simulink model "PROVA_EGO_ACC_V5"  (R2021b)
settings: Solver=ode4  StartTime=0.0  StopTime=T  FixedStep=Tc  RelTol=1e-3
values from neighbouring files (symbols this model uses):
  acc_C4 = acc_C4_all(i)    [TEST_AUTOMATICO_V1.m]
  acc_C5 = acc_C5_all(i)    [TEST_AUTOMATICO_V1.m]
  init_sim = [X0 (V0_ego_init/3.6) Angles0]'    [TEST_AUTOMATICO_V1.m]
  init_sim_C4 = [X0_C4 (V0_C4_init/3.6) Angles0_C4]'    [TEST_AUTOMATICO_V1.m]
  init_sim_C5 = [X0_C5 (V0_C5_init/3.6) Angles0_C5]'    [TEST_AUTOMATICO_V1.m]
  init_sim_C7 = [X0_C7 (V0_C7_init/3.6) Angles0_C7]'    [TEST_AUTOMATICO_V1.m]
  T = 40    [TEST_AUTOMATICO_V1.m]
  Tc = 0.1    [TEST_AUTOMATICO_V1.m]
  V0_C4_init = V0_C4(i)    [TEST_AUTOMATICO_V1.m]
  V0_C5_init = V0_C5(i)    [TEST_AUTOMATICO_V1.m]
  V0_C7_init = V0_C7(i)    [TEST_AUTOMATICO_V1.m]
  V0_ego_init = V0_ego(i)    [TEST_AUTOMATICO_V1.m]
  xx_rif = 0:Tc:x_tr(end)    [TEST_AUTOMATICO_V1.m]
  xx_rif_C4 = 0:Tc:(x_tr_C4(end))    [TEST_AUTOMATICO_V1.m]
  xx_rif_C5 = 0:Tc:(x_tr_C5(end))    [TEST_AUTOMATICO_V1.m]
  xx_rif_C7 = 0:Tc:(x_tr_C7(end))    [TEST_AUTOMATICO_V1.m]
undefined symbols (not defined in the file or in its folder): yy_rif, yy_rif_C4, yy_rif_C5, yy_rif_C7
libraries: simulink x3, mpcadaslib x2
settings Model: Creator=The MathWorks, Inc.  LastModifiedBy=NICO
settings SolverCC: AlgebraicLoopSolver=TrustRegion
settings DataIOCC: ReturnWorkspaceOutputs=off
settings DebuggingCC: SFMachineParentedDataDiag=warning  ArithmeticOperatorsInVariantConditions=warning
settings SFSimCC: SimUseLocalCustomCode=off  CustomCodeUndefinedFunction=UseInterfaceOnly
settings RTWCC: RTWUseLocalCustomCode=off
settings CodeAppCC: StateflowObjectComments=on

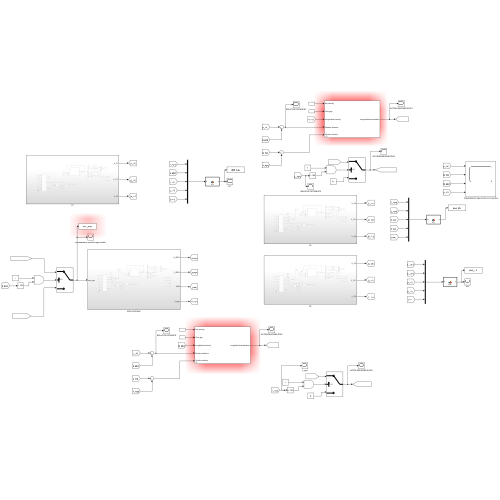
[thumbnail: Simulink's stored preview of the top-level diagram]
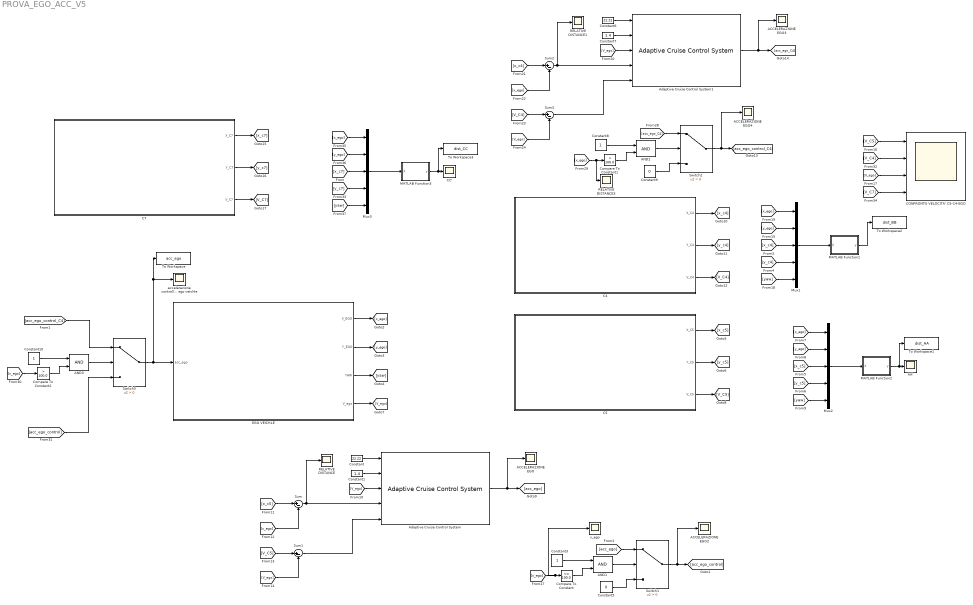
== system PROVA_EGO_ACC_V5 ==
  AA' : Scope
  ACCELERAZIONE EGO{,2..4} (4 alike) : Scope
  AND1 : Logic  IconShape=distinctive  AllPortsSameDT=off  OutDataTypeStr=boolean
  AND2 : Logic  IconShape=distinctive  AllPortsSameDT=off  OutDataTypeStr=boolean
  AND3 : Logic  IconShape=distinctive  AllPortsSameDT=off  OutDataTypeStr=boolean
  Adaptive Cruise Control System : mpcadaslib/Adaptive Cruise Control System  EgoModel=tf(1,[0.5,1,0])  InitialEgoVelocity=(V0_ego_init/3.6)  DefaultSpacing=3  MaxVelocity=22.22  MinAcceleration=-4  amin_ext=off  MaxAcceleration=2  amax_ext=off  Ts=Tc  PredictionHorizon=60  ControllerBehavior=0.380  suboptimal=off  maxiter=10  datatypeopt=double  optmode=off  trackmode=off
  Adaptive Cruise Control System1 : mpcadaslib/Adaptive Cruise Control System  EgoModel=tf(1,[0.5,1,0])  InitialEgoVelocity=(V0_C4_init/3.6)  DefaultSpacing=3  MaxVelocity=22.22  MinAcceleration=-4  amin_ext=off  MaxAcceleration=4  amax_ext=off  Ts=Tc  PredictionHorizon=30  ControllerBehavior=0.450  suboptimal=off  maxiter=10  datatypeopt=double  optmode=off  trackmode=off
  C4 : Subsystem
  C5 : Subsystem
  C7 : Subsystem
  CC' : Scope
  CONFRONTO VELOCITA' C5-C4-EGO : Scope  NumInputPorts=4
  Compare To Constant : simulink/Logic and Bit Operations/Compare To Constant  relop=<=  const=100.0  OutDataTypeStr=boolean
  Compare To Constant1 : simulink/Logic and Bit Operations/Compare To Constant  relop=>  const=100.0  OutDataTypeStr=boolean
  Compare To Constant2 : simulink/Logic and Bit Operations/Compare To Constant  relop=>  const=100.0  OutDataTypeStr=boolean
  Constant : Constant  Value=22.22
  Constant1 : Constant  Value=1.4
  Constant10 : Constant
  Constant3 : Constant
  Constant5 : Constant  Value=0
  Constant6 : Constant  Value=22.22
  Constant7 : Constant  Value=1.4
  Constant8 : Constant
  Constant9 : Constant  Value=0
  EGO VEICHLE : Subsystem
  MATLAB Function1 : MATLAB Function  TreatAsAtomicUnit=on
  MATLAB Function2 : MATLAB Function  TreatAsAtomicUnit=on
  MATLAB Function3 : MATLAB Function  TreatAsAtomicUnit=on
  Mux1 : Mux  Inputs=5
  Mux2 : Mux  Inputs=5
  Mux3 : Mux  Inputs=5
  RELATIVE DISTANCE : Scope
  RELATIVE DISTANCE1 : Scope
  RELATIVE DISTANCE3 : Scope
  Sum{,1..3} (4 alike) : Sum  Inputs=|+-
  Switch1 : Switch  Criteria=u2 > Threshold
  Switch2 : Switch  Criteria=u2 > Threshold
  Switch3 : Switch  Criteria=u2 > Threshold
  To Workspace : ToWorkspace  VariableName=acc_ego  SaveFormat=Structure With Time  SampleTime=Tc
  To Workspace1 : ToWorkspace  VariableName=dist_AA  SaveFormat=Structure With Time  SampleTime=-1
  To Workspace2 : ToWorkspace  VariableName=dist_BB  SaveFormat=Structure With Time  SampleTime=-1
  To Workspace3 : ToWorkspace  VariableName=dist_CC  SaveFormat=Structure With Time  SampleTime=-1
  accelerazione controllo ego veichle : Scope
  x_ego : Scope
  wires:
  EGO VEICHLE/1(X_EGO) -> [x_ego]
  EGO VEICHLE/2(Y_EGO) -> [y_ego]
  EGO VEICHLE/3(YAW) -> [yaw]
  C5/1(X_C5) -> [x_c5]
  C5/2("Y_C5 ") -> [y_c5]
  [x_c5] -> Mux2/3
  Mux2/1 -> MATLAB Function2/1(X)
  MATLAB Function2/1(y) -> To Workspace1/1, AA'/1
  [y_ego] -> Mux2/2
  [yaw] -> Mux2/5
  [x_ego] -> Mux2/1
  [y_c5] -> Mux2/4
  Constant/1 -> Adaptive Cruise Control System/1
  Constant1/1 -> Adaptive Cruise Control System/2
  EGO VEICHLE/4(V_ego) -> [V_ego]
  [V_ego] -> Adaptive Cruise Control System/3
  [x_c5] -> Sum/1
  [x_ego] -> Sum/2
  Sum/1 -> RELATIVE DISTANCE/1, Adaptive Cruise Control System/4
  C5/3(V_C5) -> [V_C5]
  [V_C5] -> Sum1/1
  [V_ego] -> Sum1/2
  Sum1/1 -> Adaptive Cruise Control System/5
  Adaptive Cruise Control System/1 -> [acc_ego], ACCELERAZIONE EGO/1
  [V_C5] -> CONFRONTO VELOCITA' C5-C4-EGO/1
  AND1/1 -> Switch1/2
  Switch1/1 -> [acc_ego_control], ACCELERAZIONE EGO2/1
  [x_ego] -> x_ego/1, Compare To Constant/1
  Constant5/1 -> Switch1/3
  [acc_ego] -> Switch1/1
  Constant3/1 -> AND1/1
  Compare To Constant/1 -> AND1/2
  [y_c4] -> Mux1/4
  [yaw] -> Mux1/5
  Mux1/1 -> MATLAB Function1/1(X)
  MATLAB Function1/1(y) -> To Workspace2/1
  [y_ego] -> Mux1/2
  C4/2("Y_C4 ") -> [y_c4]
  C4/1(X_C4) -> [x_c4]
  C4/3(V_C4) -> [V_C4]
  [x_c4] -> Mux1/3
  [x_ego] -> Mux1/1
  [acc_ego_C4] -> Switch2/1
  Constant9/1 -> Switch2/3
  [x_ego] -> Compare To Constant1/1, RELATIVE DISTANCE3/1
  Switch2/1 -> [acc_ego_control_C4], ACCELERAZIONE EGO4/1
  Sum3/1 -> Adaptive Cruise Control System1/5
  Compare To Constant1/1 -> AND2/2
  [x_c4] -> Sum2/1
  Constant8/1 -> AND2/1
  Constant6/1 -> Adaptive Cruise Control System1/1
  Sum2/1 -> RELATIVE DISTANCE1/1, Adaptive Cruise Control System1/4
  [V_ego] -> Adaptive Cruise Control System1/3
  AND2/1 -> Switch2/2
  [x_ego] -> Sum2/2
  [V_ego] -> Sum3/2
  [V_C4] -> Sum3/1
  Constant7/1 -> Adaptive Cruise Control System1/2
  Adaptive Cruise Control System1/1 -> [acc_ego_C4], ACCELERAZIONE EGO3/1
  AND3/1 -> Switch3/2
  Compare To Constant2/1 -> AND3/2
  [x_ego] -> Compare To Constant2/1
  Constant10/1 -> AND3/1
  [acc_ego_control_C4] -> Switch3/1
  Switch3/1 -> EGO VEICHLE/1(acc_ego), To Workspace/1, accelerazione controllo ego veichle/1
  [acc_ego_control] -> Switch3/3
  [V_C4] -> CONFRONTO VELOCITA' C5-C4-EGO/2
  [V_ego] -> CONFRONTO VELOCITA' C5-C4-EGO/3
  [y_ego] -> Mux3/2
  [yaw] -> Mux3/5
  C7/2("Y_C7 ") -> [y_c7]
  [x_ego] -> Mux3/1
  C7/3(V_C7) -> [V_C7]
  Mux3/1 -> MATLAB Function3/1(X)
  [x_c7] -> Mux3/3
  MATLAB Function3/1(y) -> To Workspace3/1, CC'/1
  C7/1(X_C7) -> [x_c7]
  [y_c7] -> Mux3/4
  [V_C7] -> CONFRONTO VELOCITA' C5-C4-EGO/4

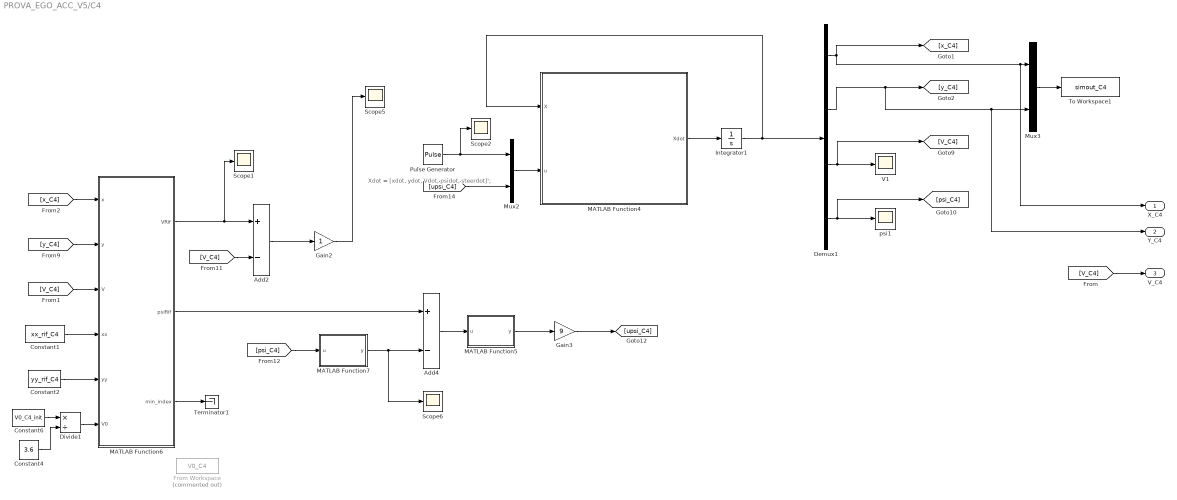
== system PROVA_EGO_ACC_V5/C4 ==
  note: Xdot = [xdot, ydot, Vdot, psidot, steerdot]';
  Add2 : Sum  Inputs=+-
  Add4 : Sum  Inputs=+-
  Constant1 : Constant  Value=xx_rif_C4
  Constant2 : Constant  Value=yy_rif_C4
  Constant4 : Constant  Value=3.6
  Constant6 : Constant  Value=V0_C4_init
  Demux1 : Demux
  Divide1 : Product  Inputs=*/
  From Workspace : FromWorkspace  Commented=on  VariableName=V0_C4
  Gain2 : Gain
  Gain3 : Gain  Gain=9
  Integrator1 : Integrator  InitialCondition=init_sim_C4
  MATLAB Function4 : MATLAB Function  TreatAsAtomicUnit=on
  MATLAB Function5 : MATLAB Function  TreatAsAtomicUnit=on
  MATLAB Function6 : MATLAB Function  TreatAsAtomicUnit=on
  MATLAB Function7 : MATLAB Function  TreatAsAtomicUnit=on
  Mux2 : Mux  Inputs=2
  Mux3 : Mux  Inputs=2
  Pulse Generator : DiscretePulseGenerator  PulseType=Time based  Amplitude=acc_C4  Period=T  PulseWidth=4
  Scope{1..2,5..6} (4 alike) : Scope
  Terminator1 : Terminator
  To Workspace1 : ToWorkspace  VariableName=simout_C4  SaveFormat=Structure With Time  SampleTime=-1
  V1 : Scope
  psi1 : Scope
  X_C4 : Outport
  "Y_C4 " : Outport  Port=2
  V_C4 : Outport  Port=3
  wires:
  Add2/1 -> Gain2/1
  [upsi_C4] -> Mux2/2
  MATLAB Function6/1(VRif) -> Scope1/1, Add2/1
  [psi_C4] -> MATLAB Function7/1(u)
  MATLAB Function7/1(y) -> Scope6/1, Add4/2
  MATLAB Function6/3(min_index) -> Terminator1/1
  Mux3/1 -> To Workspace1/1
  [x_C4] -> MATLAB Function6/1(x)
  Demux1/3 -> V1/1, [V_C4]
  MATLAB Function4/1(Xdot) -> Integrator1/1
  [V_C4] -> MATLAB Function6/3(V)
  Demux1/4 -> [psi_C4], psi1/1
  Demux1/1 -> X_C4/1, Mux3/1, [x_C4]
  Mux2/1 -> MATLAB Function4/2(u)
  Gain2/1 -> Scope5/1
  Demux1/2 -> [y_C4], "Y_C4 "/1, Mux3/2
  [y_C4] -> MATLAB Function6/2(y)
  [V_C4] -> Add2/2
  Integrator1/1 -> Demux1/1, MATLAB Function4/1(X)
  Add4/1 -> MATLAB Function5/1(u)
  Gain3/1 -> [upsi_C4]
  Constant1/1 -> MATLAB Function6/4(xx)
  MATLAB Function6/2(psiRif) -> Add4/1
  Constant2/1 -> MATLAB Function6/5(yy)
  MATLAB Function5/1(y) -> Gain3/1
  [V_C4] -> V_C4/1
  Pulse Generator/1 -> Scope2/1, Mux2/1
  Constant4/1 -> Divide1/2
  Constant6/1 -> Divide1/1
  Divide1/1 -> MATLAB Function6/6(V0)

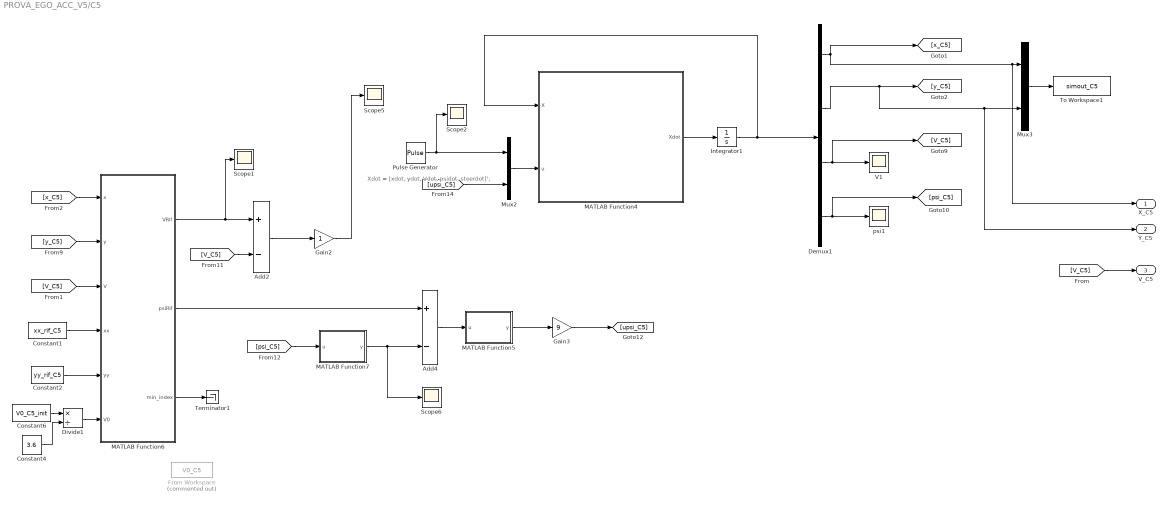
== system PROVA_EGO_ACC_V5/C5 ==
  note: Xdot = [xdot, ydot, Vdot, psidot, steerdot]';
  Add2 : Sum  Inputs=+-
  Add4 : Sum  Inputs=+-
  Constant1 : Constant  Value=xx_rif_C5
  Constant2 : Constant  Value=yy_rif_C5
  Constant4 : Constant  Value=3.6
  Constant6 : Constant  Value=V0_C5_init
  Demux1 : Demux
  Divide1 : Product  Inputs=*/
  From Workspace : FromWorkspace  Commented=on  VariableName=V0_C5  SampleTime=Tc
  Gain2 : Gain
  Gain3 : Gain  Gain=9
  Integrator1 : Integrator  InitialCondition=init_sim_C5
  MATLAB Function4 : MATLAB Function  TreatAsAtomicUnit=on
  MATLAB Function5 : MATLAB Function  TreatAsAtomicUnit=on
  MATLAB Function6 : MATLAB Function  TreatAsAtomicUnit=on
  MATLAB Function7 : MATLAB Function  TreatAsAtomicUnit=on
  Mux2 : Mux  Inputs=2
  Mux3 : Mux  Inputs=2
  Pulse Generator : DiscretePulseGenerator  PulseType=Time based  Amplitude=acc_C5  Period=T  PulseWidth=6
  Scope{1..2,5..6} (4 alike) : Scope
  Terminator1 : Terminator
  To Workspace1 : ToWorkspace  VariableName=simout_C5  SaveFormat=Structure With Time  SampleTime=-1
  V1 : Scope
  psi1 : Scope
  X_C5 : Outport
  "Y_C5 " : Outport  Port=2
  V_C5 : Outport  Port=3
  wires:
  Add2/1 -> Gain2/1
  [upsi_C5] -> Mux2/2
  MATLAB Function6/1(VRif) -> Scope1/1, Add2/1
  [psi_C5] -> MATLAB Function7/1(u)
  MATLAB Function7/1(y) -> Scope6/1, Add4/2
  MATLAB Function6/3(min_index) -> Terminator1/1
  Mux3/1 -> To Workspace1/1
  [x_C5] -> MATLAB Function6/1(x)
  Demux1/3 -> V1/1, [V_C5]
  MATLAB Function4/1(Xdot) -> Integrator1/1
  [V_C5] -> MATLAB Function6/3(V)
  Demux1/4 -> [psi_C5], psi1/1
  Demux1/1 -> X_C5/1, Mux3/1, [x_C5]
  Mux2/1 -> MATLAB Function4/2(u)
  Gain2/1 -> Scope5/1
  Demux1/2 -> [y_C5], "Y_C5 "/1, Mux3/2
  [y_C5] -> MATLAB Function6/2(y)
  [V_C5] -> Add2/2
  Integrator1/1 -> Demux1/1, MATLAB Function4/1(X)
  Add4/1 -> MATLAB Function5/1(u)
  Gain3/1 -> [upsi_C5]
  Constant1/1 -> MATLAB Function6/4(xx)
  MATLAB Function6/2(psiRif) -> Add4/1
  Constant2/1 -> MATLAB Function6/5(yy)
  MATLAB Function5/1(y) -> Gain3/1
  [V_C5] -> V_C5/1
  Pulse Generator/1 -> Mux2/1, Scope2/1
  Constant4/1 -> Divide1/2
  Constant6/1 -> Divide1/1
  Divide1/1 -> MATLAB Function6/6(V0)

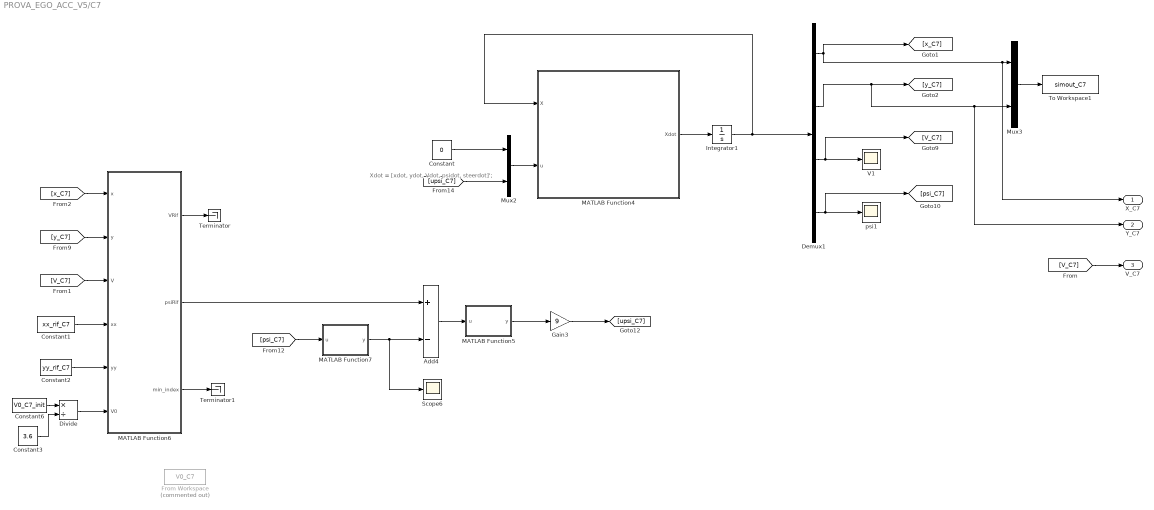
== system PROVA_EGO_ACC_V5/C7 ==
  note: Xdot = [xdot, ydot, Vdot, psidot, steerdot]';
  Add4 : Sum  Inputs=+-
  Constant : Constant  Value=0
  Constant1 : Constant  Value=xx_rif_C7
  Constant2 : Constant  Value=yy_rif_C7
  Constant3 : Constant  Value=3.6
  Constant6 : Constant  Value=V0_C7_init
  Demux1 : Demux
  Divide : Product  Inputs=*/
  From Workspace : FromWorkspace  Commented=on  VariableName=V0_C7  SampleTime=Tc
  Gain3 : Gain  Gain=9
  Integrator1 : Integrator  InitialCondition=init_sim_C7
  MATLAB Function4 : MATLAB Function  TreatAsAtomicUnit=on
  MATLAB Function5 : MATLAB Function  TreatAsAtomicUnit=on
  MATLAB Function6 : MATLAB Function  TreatAsAtomicUnit=on
  MATLAB Function7 : MATLAB Function  TreatAsAtomicUnit=on
  Mux2 : Mux  Inputs=2
  Mux3 : Mux  Inputs=2
  Scope6 : Scope
  Terminator : Terminator
  Terminator1 : Terminator
  To Workspace1 : ToWorkspace  VariableName=simout_C7  SaveFormat=Structure With Time  SampleTime=-1
  V1 : Scope
  psi1 : Scope
  X_C7 : Outport
  "Y_C7 " : Outport  Port=2
  V_C7 : Outport  Port=3
  wires:
  [upsi_C7] -> Mux2/2
  [psi_C7] -> MATLAB Function7/1(u)
  MATLAB Function7/1(y) -> Scope6/1, Add4/2
  MATLAB Function6/3(min_index) -> Terminator1/1
  Mux3/1 -> To Workspace1/1
  [x_C7] -> MATLAB Function6/1(x)
  Demux1/3 -> V1/1, [V_C7]
  MATLAB Function4/1(Xdot) -> Integrator1/1
  [V_C7] -> MATLAB Function6/3(V)
  Demux1/4 -> [psi_C7], psi1/1
  Demux1/1 -> X_C7/1, Mux3/1, [x_C7]
  Mux2/1 -> MATLAB Function4/2(u)
  Demux1/2 -> [y_C7], "Y_C7 "/1, Mux3/2
  [y_C7] -> MATLAB Function6/2(y)
  Integrator1/1 -> Demux1/1, MATLAB Function4/1(X)
  Add4/1 -> MATLAB Function5/1(u)
  Gain3/1 -> [upsi_C7]
  Constant1/1 -> MATLAB Function6/4(xx)
  MATLAB Function6/2(psiRif) -> Add4/1
  Constant2/1 -> MATLAB Function6/5(yy)
  MATLAB Function5/1(y) -> Gain3/1
  [V_C7] -> V_C7/1
  MATLAB Function6/1(VRif) -> Terminator/1
  Constant/1 -> Mux2/1
  Constant6/1 -> Divide/1
  Divide/1 -> MATLAB Function6/6(V0)
  Constant3/1 -> Divide/2

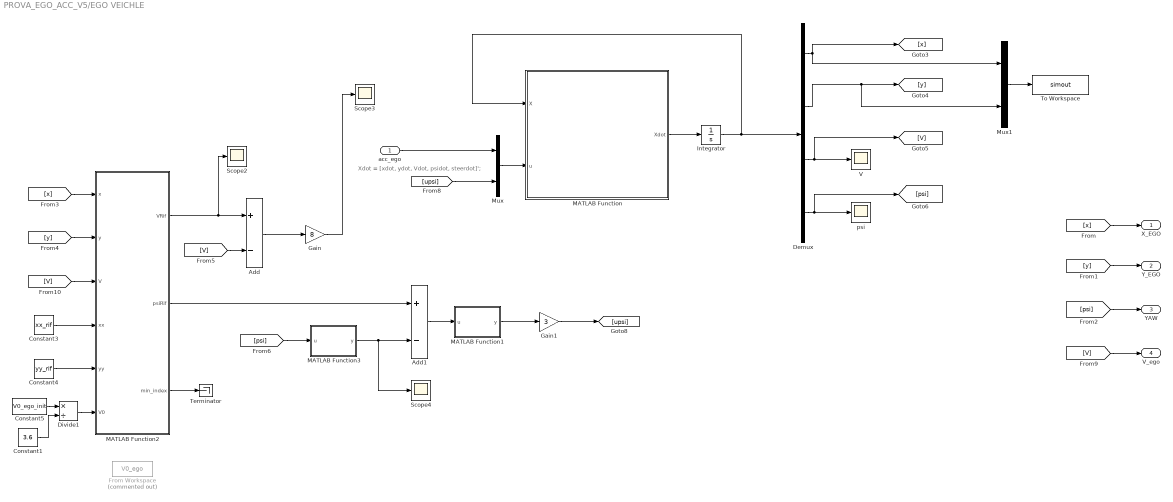
== system PROVA_EGO_ACC_V5/EGO VEICHLE ==
  note: Xdot = [xdot, ydot, Vdot, psidot, steerdot]';
  acc_ego : Inport
  Add : Sum  Inputs=+-
  Add1 : Sum  Inputs=+-
  Constant1 : Constant  Value=3.6
  Constant3 : Constant  Value=xx_rif
  Constant4 : Constant  Value=yy_rif
  Constant5 : Constant  Value=V0_ego_init
  Demux : Demux
  Divide1 : Product  Inputs=*/
  From Workspace : FromWorkspace  Commented=on  VariableName=V0_ego  SampleTime=Tc
  Gain : Gain  Gain=8
  Gain1 : Gain  Gain=3
  Integrator : Integrator  InitialCondition=init_sim
  MATLAB Function : MATLAB Function  TreatAsAtomicUnit=on
  MATLAB Function1 : MATLAB Function  TreatAsAtomicUnit=on
  MATLAB Function2 : MATLAB Function  TreatAsAtomicUnit=on
  MATLAB Function3 : MATLAB Function  TreatAsAtomicUnit=on
  Mux : Mux  Inputs=2
  Mux1 : Mux  Inputs=2
  Scope2 : Scope
  Scope3 : Scope
  Scope4 : Scope
  Terminator : Terminator
  To Workspace : ToWorkspace  VariableName=simout  SaveFormat=Structure With Time  SampleTime=-1
  V : Scope
  psi : Scope
  X_EGO : Outport
  Y_EGO : Outport  Port=2
  YAW : Outport  Port=3
  V_ego : Outport  Port=4
  wires:
  Constant4/1 -> MATLAB Function2/5(yy)
  Demux/1 -> Mux1/1, [x]
  [upsi] -> Mux/2
  MATLAB Function3/1(y) -> Scope4/1, Add1/2
  MATLAB Function2/1(VRif) -> Scope2/1, Add/1
  Integrator/1 -> Demux/1, MATLAB Function/1(X)
  [V] -> MATLAB Function2/3(V)
  Gain1/1 -> [upsi]
  MATLAB Function2/3(min_index) -> Terminator/1
  Demux/4 -> [psi], psi/1
  Constant3/1 -> MATLAB Function2/4(xx)
  Gain/1 -> Scope3/1
  Demux/2 -> [y], Mux1/2
  Demux/3 -> V/1, [V]
  [y] -> MATLAB Function2/2(y)
  Mux/1 -> MATLAB Function/2(u)
  MATLAB Function/1(Xdot) -> Integrator/1
  acc_ego/1 -> Mux/1
  Add/1 -> Gain/1
  [x] -> MATLAB Function2/1(x)
  Mux1/1 -> To Workspace/1
  MATLAB Function1/1(y) -> Gain1/1
  MATLAB Function2/2(psiRif) -> Add1/1
  [psi] -> MATLAB Function3/1(u)
  [V] -> Add/2
  Add1/1 -> MATLAB Function1/1(u)
  [x] -> X_EGO/1
  [y] -> Y_EGO/1
  [psi] -> YAW/1
  [V] -> V_ego/1
  Constant1/1 -> Divide1/2
  Constant5/1 -> Divide1/1
  Divide1/1 -> MATLAB Function2/6(V0)

== matlab function PROVA_EGO_ACC_V5/C5/MATLAB Function5 ==
  data: u input; y output
function y = wrapPi(u)
y = wrap_Pi(u);
end

== matlab function PROVA_EGO_ACC_V5/C5/MATLAB Function6 ==
  data: x input; VRif output; y input; V input; xx input; yy input; V0 input; psiRif output; min_index output
function [VRif,psiRif,min_index] = pathfollower_mono(x, y, V, xx, yy,V0)

n = length(xx);
d_ref = zeros(1,n);

for i = 1:n
d_ref(i)= sqrt((xx(i)-x)^2+(yy(i)-y)^2);
end

[~, min_index] = min(d_ref);

m = length(V0)
for j = 1:m
   if d_ref(end)<0.1     %%% errore di riferimento
     VRif=0;
   else
    VRif=V0(j);
   end
end


% if d_ref(end)<0.1     %%% errore di riferimento
% VRif=0;
% else
% VRif=V0;
% end

min_index = min(min_index + 1, n);                                  %%% per dargli una curva più smooth gli do qualche punto più avanti invece di quello attuale
psiRif = wrap_2Pi(atan2((yy(min_index)-y),(xx(min_index)-x)));

end

== matlab function PROVA_EGO_ACC_V5/C5/MATLAB Function7 ==
  data: u input; y output
function y = wrap2Pi(u)
y = wrap_2Pi(u);
end

== matlab function PROVA_EGO_ACC_V5/MATLAB Function2 ==
  data: X input; y output
function y = fcn(X)

w_ego = 1.8 ; % larghezza auto ego
w_C4 = 1.8 ; % larghezza auto C7

a = 2 ; % semi-lunghezza ego
b = 2 ; % semi-lunghezza C7

x0 = X(1) ;
y0 = X(2) ;

x_C5 = X(3) ;
y_C5 = X(4) ;

theta = X(5) ;

u = sqrt(  (x0 + a*cos(theta) + (1/2)*w_ego*sin(theta) - x_C5 + b )^2  + ...
           (y0 + a*sin(theta) - (1/2)*w_ego*cos(theta) - y_C5 - (1/2)*w_C4)^2   )

y = u;

== matlab function PROVA_EGO_ACC_V5/C7/MATLAB Function4 ==
  data: X input; u input; Xdot output
function Xdot = fcn(X,u)

L = 2.5;

x = X(1);
y = X(2);
V = X(3);
psi = X(4);                  %%% imbardata
% steer = X(5);

xdot = V*cos(psi);
ydot = V*sin(psi);
Vdot = u(1);                 %%% non ci sono variazioni del modulo della velocità
psidot = u(2);

% psidot = (V/L)*tan(steer);  
% steerdot = u(2);

% Xdot = [xdot, ydot, Vdot, psidot, steerdot]';
Xdot = [xdot, ydot, Vdot, psidot]';

end

== matlab function PROVA_EGO_ACC_V5/EGO VEICHLE/MATLAB Function1 ==
  data: u input; y output
function y = wrapPi(u)
y = wrap_Pi(u);
end

== matlab function PROVA_EGO_ACC_V5/C7/MATLAB Function5 ==
  data: u input; y output
function y = wrapPi(u)
y = wrap_Pi(u);
end

== matlab function PROVA_EGO_ACC_V5/C7/MATLAB Function6 ==
  data: x input; VRif output; y input; V input; xx input; yy input; V0 input; psiRif output; min_index output
function [VRif,psiRif,min_index] = pathfollower_mono(x, y, V, xx, yy,V0)

n = length(xx);
d_ref = zeros(1,n);

for i = 1:n
d_ref(i)= sqrt((xx(i)-x)^2+(yy(i)-y)^2);
end

[~, min_index] = min(d_ref);

m = length(V0)
for j = 1:m
   if d_ref(end)<0.1     %%% errore di riferimento
     VRif=0;
   else
    VRif=V0(j);
   end
end


% if d_ref(end)<0.1     %%% errore di riferimento
% VRif=0;
% else
% VRif=V0;
% end

min_index = min(min_index + 1, n);                                  %%% per dargli una curva più smooth gli do qualche punto più avanti invece di quello attuale
psiRif = wrap_2Pi(atan2((yy(min_index)-y),(xx(min_index)-x)));

end

== matlab function PROVA_EGO_ACC_V5/C7/MATLAB Function7 ==
  data: u input; y output
function y = wrap2Pi(u)
y = wrap_2Pi(u);
end

== matlab function PROVA_EGO_ACC_V5/MATLAB Function3 ==
  data: X input; y output
function y = fcn(X)

w_ego = 1.8 ; % larghezza auto ego
w_C7 = 1.8 ; % larghezza auto C7

a = 2 ; % semi-lunghezza ego
b = 2 ; % semi-lunghezza C7

x0 = X(1) ;
y0 = X(2) ;

x_C7 = X(3) ;
y_C7 = X(4) ;

theta = X(5) ;

u = sqrt(  (x0 - a*cos(theta) - (1/2)*w_ego*sin(theta) - x_C7 - b )^2  + ...
           (y0 - a*sin(theta) + (1/2)*w_ego*cos(theta) - y_C7 + (1/2)*w_C7)^2   )

y = u;

== matlab function PROVA_EGO_ACC_V5/EGO VEICHLE/MATLAB Function ==
  data: X input; u input; Xdot output
function Xdot = fcn(X,u)

L = 2.5;

x = X(1);
y = X(2);
V = X(3);
psi = X(4);                  %%% imbardata
% steer = X(5);

xdot = V*cos(psi);
ydot = V*sin(psi);
Vdot = u(1);                 %%% non ci sono variazioni del modulo della velocità
psidot = u(2);

% psidot = (V/L)*tan(steer);  
% steerdot = u(2);

% Xdot = [xdot, ydot, Vdot, psidot, steerdot]';
Xdot = [xdot, ydot, Vdot, psidot]';

end

== matlab function PROVA_EGO_ACC_V5/EGO VEICHLE/MATLAB Function2 ==
  data: x input; VRif output; y input; V input; xx input; yy input; V0 input; psiRif output; min_index output
function [VRif,psiRif,min_index] = pathfollower_mono(x, y, V, xx, yy,V0)

n = length(xx);
d_ref = zeros(1,n);

for i = 1:n
d_ref(i)= sqrt((xx(i)-x)^2+(yy(i)-y)^2);
end

[~, min_index] = min(d_ref);

m = length(V0)
for j = 1:m
   if d_ref(end)<0.1     %%% errore di riferimento
     VRif=0;
   else
    VRif=V0(j);
   end
end


% if d_ref(end)<0.1     %%% errore di riferimento
% VRif=0;
% else
% VRif=V0;
% end

min_index = min(min_index + 1, n);                                  %%% per dargli una curva più smooth gli do qualche punto più avanti invece di quello attuale
psiRif = wrap_2Pi(atan2((yy(min_index)-y),(xx(min_index)-x)));

end

== matlab function PROVA_EGO_ACC_V5/C4/MATLAB Function4 ==
  data: X input; u input; Xdot output
function Xdot = fcn(X,u)

L = 2.5;

x = X(1);
y = X(2);
V = X(3);
psi = X(4);                  %%% imbardata
% steer = X(5);

xdot = V*cos(psi);
ydot = V*sin(psi);
Vdot = u(1);                 %%% non ci sono variazioni del modulo della velocità
psidot = u(2);

% psidot = (V/L)*tan(steer);  
% steerdot = u(2);

% Xdot = [xdot, ydot, Vdot, psidot, steerdot]';
Xdot = [xdot, ydot, Vdot, psidot]';

end

== matlab function PROVA_EGO_ACC_V5/EGO VEICHLE/MATLAB Function3 ==
  data: u input; y output
function y = wrap2Pi(u)
y = wrap_2Pi(u);
end

== matlab function PROVA_EGO_ACC_V5/C4/MATLAB Function5 ==
  data: u input; y output
function y = wrapPi(u)
y = wrap_Pi(u);
end

== matlab function PROVA_EGO_ACC_V5/C4/MATLAB Function6 ==
  data: x input; VRif output; y input; V input; xx input; yy input; V0 input; psiRif output; min_index output
function [VRif,psiRif,min_index] = pathfollower_mono(x, y, V, xx, yy,V0)

n = length(xx);
d_ref = zeros(1,n);

for i = 1:n
d_ref(i)= sqrt((xx(i)-x)^2+(yy(i)-y)^2);
end

[~, min_index] = min(d_ref);

m = length(V0)
for j = 1:m
   if d_ref(end)<0.1     %%% errore di riferimento
     VRif=0;
   else
    VRif=V0(j);
   end
end


% if d_ref(end)<0.1     %%% errore di riferimento
% VRif=0;
% else
% VRif=V0;
% end

min_index = min(min_index + 1, n);                                  %%% per dargli una curva più smooth gli do qualche punto più avanti invece di quello attuale
psiRif = wrap_2Pi(atan2((yy(min_index)-y),(xx(min_index)-x)));

end

== matlab function PROVA_EGO_ACC_V5/C4/MATLAB Function7 ==
  data: u input; y output
function y = wrap2Pi(u)
y = wrap_2Pi(u);
end

== matlab function PROVA_EGO_ACC_V5/MATLAB Function1 ==
  data: X input; y output
function y = fcn(X)

w_ego = 1.8 ; % larghezza auto ego
w_C4 = 1.8 ; % larghezza auto C7

a = 2 ; % semi-lunghezza ego
b = 2 ; % semi-lunghezza C7

x0 = X(1) ;
y0 = X(2) ;

x_C4 = X(3) ;
y_C4 = X(4) ;

theta = X(5) ;

u = sqrt(  (x0 + a*cos(theta) - (1/2)*w_ego*sin(theta) - x_C4 + b )^2  + ...
           (y0 + a*sin(theta) + (1/2)*w_ego*cos(theta) - y_C4 + (1/2)*w_C4)^2   )

y = u;

== matlab function PROVA_EGO_ACC_V5/C5/MATLAB Function4 ==
  data: X input; u input; Xdot output
function Xdot = fcn(X,u)

L = 2.5;

x = X(1);
y = X(2);
V = X(3);
psi = X(4);                  %%% imbardata
% steer = X(5);

xdot = V*cos(psi);
ydot = V*sin(psi);
Vdot = u(1);                 %%% non ci sono variazioni del modulo della velocità
psidot = u(2);

% psidot = (V/L)*tan(steer);  
% steerdot = u(2);

% Xdot = [xdot, ydot, Vdot, psidot, steerdot]';
Xdot = [xdot, ydot, Vdot, psidot]';

end
